simulink model "MdXXArray"  (R2024b)
settings: Solver=FixedStepDiscrete  StartTime=0.0  StopTime=10.0  FixedStep=0.01  RelTol=1e-3
(part 1 of 2)
settings Model: Creator=sn2xws  LastModifiedBy=sn55gm
settings Model: ModifiedHistory=|
  | 2023.8.1 V2.0.0 CR401790 增加模式21-26
  | 2024.7.12 V3.0.0  557模式流程V1.9
  | 2024.10.15 V3.0.1 新增Md57 58
  | 25.6.27 V3.13.0 新增Md62 Md61
settings SolverCC: AlgebraicLoopSolver=TrustRegion
settings DataIOCC: SaveFormat=StructureWithTime  ReturnWorkspaceOutputs=off
settings OptimizationCC: DefaultParameterBehavior=Inlined  EnhancedBackFolding=on  PassReuseOutputArgsAs=Individual arguments  ZeroExternalMemoryAtStartup=off  ZeroInternalMemoryAtStartup=off  OptimizeBlockOrder=speed  DifferentSizesBufferReuse=on  OptimizationCustomize=off  EfficientTunableParamExpr=on
settings DebuggingCC: ParameterTunabilityLossMsg=error  UnconnectedInputMsg=warning  UnconnectedOutputMsg=warning  UnconnectedLineMsg=warning  ArithmeticOperatorsInVariantConditions=warning
settings ModelReferenceCC: EnableRefExpFcnMdlSchedulingChecks=on
settings SFSimCC: MATLABDynamicMemAlloc=off  CustomCodeUndefinedFunction=UseInterfaceOnly
settings RTWCC: Description=AUTOSAR  SystemTargetFile=autosar.tlc  GenCodeOnly=on  TemplateMakefile=ert_default_tmf  GenerateReport=on  IncludeHyperlinkInReport=on  LaunchReport=on  DataTypeReplacement=CDataTypesFixedWidth  GenerateTraceInfo=on  GenerateTraceReport=on  GenerateTraceReportSl=on  GenerateTraceReportSf=on  GenerateTraceReportEml=on  GenerateCodeMetricsReport=on  GPUComputeCapability=3.5
settings CodeAppCC: ForceParamTrailComments=on  IgnoreCustomStorageClasses=off  OperatorAnnotations=on  SimulinkDataObjDesc=on  SFDataObjDesc=on  InsertBlockDesc=on
settings STFCustomTargetCC: TargetLangStandard=C99 (ISO)  MultiwordLength=256  ParMdlRefBuildCompliant=on  CompOptLevelCompliant=on  IncludeMdlTerminateFcn=off  CombineOutputUpdateFcns=on  SuppressErrorStatus=on  ERTCustomFileBanners=on  SupportNonFinite=off  SupportComplex=off  SupportContinuousTime=off  SupportNonInlinedSFcns=off  RemoveResetFunc=on  MATLABClassNameForMDSCustomization=Simulink.SoftwareTarget.ERTCustomization  AutosarCompliant=on  UseToolchainInfoCompliant=on  LookupTableObjectStructAxisOrder=2,1,3,4,...  LUTObjectStructOrderEvenSpacing=Size,Table,Breakpoints  SystemTargetFile=autosar.tlc
settings ERTTargetCC: TargetLangStandard=C99 (ISO)  ConcurrentExecutionCompliant=off  IncludeMdlTerminateFcn=off  SuppressErrorStatus=on  SupportNonFinite=off  SupportComplex=off  ModelStepFunctionPrototypeControlCompliant=off  CPPClassGenCompliant=off  AutosarCompliant=on  LookupTableObjectStructAxisOrder=2,1,3,4,...  LUTObjectStructOrderEvenSpacing=Size,Table,Breakpoints  ERTCustomFileTemplate=example_file_process.tlc  ERTFilePackagingFormat=Compact  BooleanTrueId=TRUE  BooleanFalseId=FALSE  DynamicArrayContainerType=coder::array

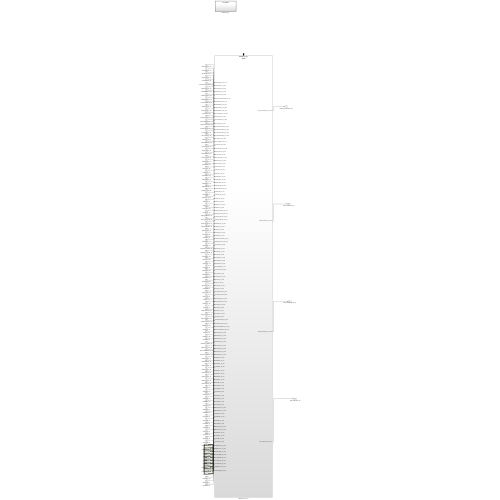
[thumbnail: Simulink's stored preview of the top-level diagram]
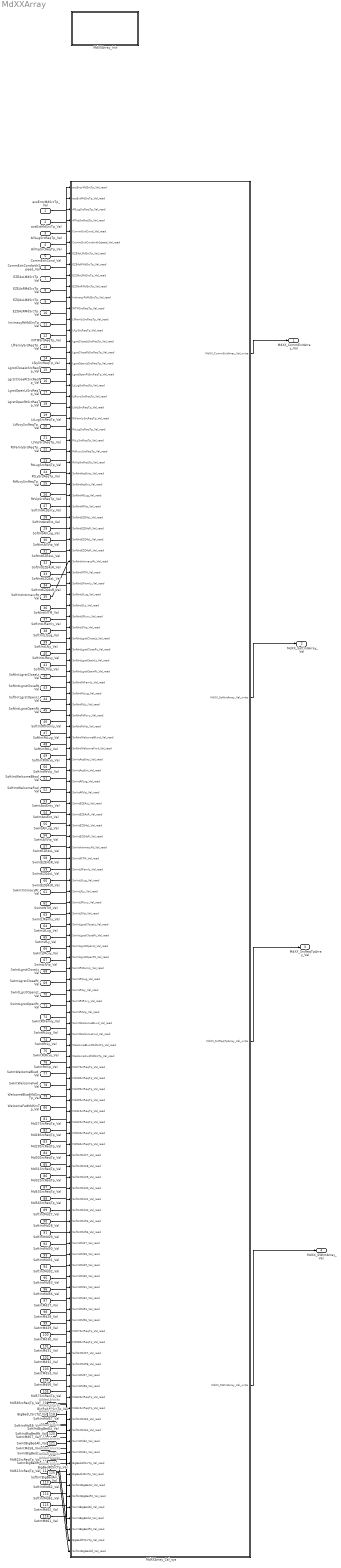
== system MdXXArray ==
  note: Added blocks
  note: Added blocks
  note: Added blocks
  note: Added blocks
  note: Added blocks
  note: Added blocks
  note: Added blocks
  note: Added blocks
  note: Added blocks
  acsEntyMdSrcTp_Val : Inport  OutDataTypeStr=Enum: SrcReqTp1  PortDimensions=1
  acsExtMdSrcTp_Val : Inport  Port=2  OutDataTypeStr=Enum: SrcReqTp1  PortDimensions=1
  AllLugSrcReqTp_Val : Inport  Port=3  OutDataTypeStr=Enum: SrcReqTp1  PortDimensions=1
  AllVipSrcReqTp_Val : Inport  Port=4  OutDataTypeStr=Enum: SrcReqTp1  PortDimensions=1
  CommExitCond_Val : Inport  Port=5  OutDataTypeStr=boolean  PortDimensions=1
  CommExitCondwithSpeed_Val : Inport  Port=6  OutDataTypeStr=boolean  PortDimensions=1
  EZE4sLMdSrcTp_Val : Inport  Port=7  OutDataTypeStr=Enum: SrcReqTp1  PortDimensions=1
  EZE4sRMdSrcTp_Val : Inport  Port=8  OutDataTypeStr=Enum: SrcReqTp1  PortDimensions=1
  EZQ4sLMdSrcTp_Val : Inport  Port=9  OutDataTypeStr=Enum: SrcReqTp1  PortDimensions=1
  EZQ4sRMdSrcTp_Val : Inport  Port=10  OutDataTypeStr=Enum: SrcReqTp1  PortDimensions=1
  IntimacyRtMdSrcTp_Val : Inport  Port=11  OutDataTypeStr=Enum: SrcReqTp1  PortDimensions=1
  INTMSrcReqTp_Val : Inport  Port=12  OutDataTypeStr=Enum: SrcReqTp1  PortDimensions=1
  LfFamlySrcReqTp_Val : Inport  Port=13  OutDataTypeStr=Enum: SrcReqTp1  PortDimensions=1
  LfLySrcReqTp_Val : Inport  Port=14  OutDataTypeStr=Enum: SrcReqTp1  PortDimensions=1
  LgrstCloseLtSrcReqTp_Val : Inport  Port=15  OutDataTypeStr=Enum: SrcReqTp1  PortDimensions=1
  LgrstCloseRtSrcReqTp_Val : Inport  Port=16  OutDataTypeStr=Enum: SrcReqTp1  PortDimensions=1
  LgrstOpenLtSrcReqTp_Val : Inport  Port=17  OutDataTypeStr=Enum: SrcReqTp1  PortDimensions=1
  LgrstOpenRtSrcReqTp_Val : Inport  Port=18  OutDataTypeStr=Enum: SrcReqTp1  PortDimensions=1
  LtLugSrcReqTp_Val : Inport  Port=19  OutDataTypeStr=Enum: SrcReqTp1  PortDimensions=1
  LtRcvySrcReqTp_Val : Inport  Port=20  OutDataTypeStr=Enum: SrcReqTp1  PortDimensions=1
  LtVipSrcReqTp_Val : Inport  Port=21  OutDataTypeStr=Enum: SrcReqTp1  PortDimensions=1
  RtFamlySrcReqTp_Val : Inport  Port=22  OutDataTypeStr=Enum: SrcReqTp1  PortDimensions=1
  RtLugSrcReqTp_Val : Inport  Port=23  OutDataTypeStr=Enum: SrcReqTp1  PortDimensions=1
  RtLySrcReqTp_Val : Inport  Port=24  OutDataTypeStr=Enum: SrcReqTp1  PortDimensions=1
  RtRcvySrcReqTp_Val : Inport  Port=25  OutDataTypeStr=Enum: SrcReqTp1  PortDimensions=1
  RtVipSrcReqTp_Val : Inport  Port=26  OutDataTypeStr=Enum: SrcReqTp1  PortDimensions=1
  SoftIntAcsEnty_Val : Inport  Port=27  OutDataTypeStr=IntEnable  PortDimensions=1
  SoftIntAcsExt_Val : Inport  Port=28  OutDataTypeStr=IntEnable  PortDimensions=1
  SoftIntAllLug_Val : Inport  Port=29  OutDataTypeStr=IntEnable  PortDimensions=1
  SoftIntAllVip_Val : Inport  Port=30  OutDataTypeStr=IntEnable  PortDimensions=1
  SoftIntEZE4sL_Val : Inport  Port=31  OutDataTypeStr=IntEnable  PortDimensions=1
  SoftIntEZE4sR_Val : Inport  Port=32  OutDataTypeStr=IntEnable  PortDimensions=1
  SoftIntEZQ4sL_Val : Inport  Port=33  OutDataTypeStr=IntEnable  PortDimensions=1
  SoftIntEZQ4sR_Val : Inport  Port=34  OutDataTypeStr=IntEnable  PortDimensions=1
  SoftIntIntimacyRt_Val : Inport  Port=35  OutDataTypeStr=IntEnable  PortDimensions=1
  SoftIntINTM_Val : Inport  Port=36  OutDataTypeStr=IntEnable  PortDimensions=1
  SoftIntLfFamly_Val : Inport  Port=37  OutDataTypeStr=IntEnable  PortDimensions=1
  SoftIntLfLug_Val : Inport  Port=38  OutDataTypeStr=IntEnable  PortDimensions=1
  SoftIntLfLy_Val : Inport  Port=39  OutDataTypeStr=IntEnable  PortDimensions=1
  SoftIntLfRcvy_Val : Inport  Port=40  OutDataTypeStr=IntEnable  PortDimensions=1
  SoftIntLfVip_Val : Inport  Port=41  OutDataTypeStr=IntEnable  PortDimensions=1
  SoftIntLgrstCloseLt_Val : Inport  Port=42  OutDataTypeStr=IntEnable  PortDimensions=1
  SoftIntLgrstCloseRt_Val : Inport  Port=43  OutDataTypeStr=IntEnable  PortDimensions=1
  SoftIntLgrstOpenLt_Val : Inport  Port=44  OutDataTypeStr=IntEnable  PortDimensions=1
  SoftIntLgrstOpenRt_Val : Inport  Port=45  OutDataTypeStr=IntEnable  PortDimensions=1
  SoftIntRtFamly_Val : Inport  Port=46  OutDataTypeStr=IntEnable  PortDimensions=1
  SoftIntRtLug_Val : Inport  Port=47  OutDataTypeStr=IntEnable  PortDimensions=1
  SoftIntRtLy_Val : Inport  Port=48  OutDataTypeStr=IntEnable  PortDimensions=1
  SoftIntRtRcvy_Val : Inport  Port=49  OutDataTypeStr=IntEnable  PortDimensions=1
  SoftIntRtVip_Val : Inport  Port=50  OutDataTypeStr=IntEnable  PortDimensions=1
  SoftIntWelcomeBkwd_Val : Inport  Port=51  OutDataTypeStr=IntEnable  PortDimensions=1
  SoftIntWelcomeFwd_Val : Inport  Port=52  OutDataTypeStr=IntEnable  PortDimensions=1
  SwIntAcsEnty_Val : Inport  Port=53  OutDataTypeStr=IntEnable  PortDimensions=1
  SwIntAcsExt_Val : Inport  Port=54  OutDataTypeStr=IntEnable  PortDimensions=1
  SwIntAllLug_Val : Inport  Port=55  OutDataTypeStr=IntEnable  PortDimensions=1
  SwIntAllVip_Val : Inport  Port=56  OutDataTypeStr=IntEnable  PortDimensions=1
  SwIntEZE4sL_Val : Inport  Port=57  OutDataTypeStr=IntEnable  PortDimensions=1
  SwIntEZE4sR_Val : Inport  Port=58  OutDataTypeStr=IntEnable  PortDimensions=1
  SwIntEZQ4sL_Val : Inport  Port=59  OutDataTypeStr=IntEnable  PortDimensions=1
  SwIntEZQ4sR_Val : Inport  Port=60  OutDataTypeStr=IntEnable  PortDimensions=1
  SwIntIntimacyRt_Val : Inport  Port=61  OutDataTypeStr=IntEnable  PortDimensions=1
  SwIntINTM_Val : Inport  Port=62  OutDataTypeStr=IntEnable  PortDimensions=1
  SwIntLfFamly_Val : Inport  Port=63  OutDataTypeStr=IntEnable  PortDimensions=1
  SwIntLfLug_Val : Inport  Port=64  OutDataTypeStr=IntEnable  PortDimensions=1
  SwIntLfLy_Val : Inport  Port=65  OutDataTypeStr=IntEnable  PortDimensions=1
  SwIntLfRcvy_Val : Inport  Port=66  OutDataTypeStr=IntEnable  PortDimensions=1
  SwIntLfVip_Val : Inport  Port=67  OutDataTypeStr=IntEnable  PortDimensions=1
  SwIntLgrstCloseLt_Val : Inport  Port=68  OutDataTypeStr=IntEnable  PortDimensions=1
  SwIntLgrstCloseRt_Val : Inport  Port=69  OutDataTypeStr=IntEnable  PortDimensions=1
  SwIntLgrstOpenLt_Val : Inport  Port=70  OutDataTypeStr=IntEnable  PortDimensions=1
  SwIntLgrstOpenRt_Val : Inport  Port=71  OutDataTypeStr=IntEnable  PortDimensions=1
  SwIntRtFamly_Val : Inport  Port=72  OutDataTypeStr=IntEnable  PortDimensions=1
  SwIntRtLug_Val : Inport  Port=73  OutDataTypeStr=IntEnable  PortDimensions=1
  SwIntRtLy_Val : Inport  Port=74  OutDataTypeStr=IntEnable  PortDimensions=1
  SwIntRtRcvy_Val : Inport  Port=75  OutDataTypeStr=IntEnable  PortDimensions=1
  SwIntRtVip_Val : Inport  Port=76  OutDataTypeStr=IntEnable  PortDimensions=1
  SwIntWelcomeBkwd_Val : Inport  Port=77  OutDataTypeStr=IntEnable  PortDimensions=1
  SwIntWelcomeFwd_Val : Inport  Port=78  OutDataTypeStr=IntEnable  PortDimensions=1
  WelcomeBkwdMdSrcTp_Val : Inport  Port=79  OutDataTypeStr=Enum: SrcReqTp1  PortDimensions=1
  WelcomeFwdMdSrcTp_Val : Inport  Port=80  OutDataTypeStr=Enum: SrcReqTp1  PortDimensions=1
  Md27SrcReqTp_Val : Inport  Port=81  OutDataTypeStr=Enum: SrcReqTp1  PortDimensions=1
  Md28SrcReqTp_Val : Inport  Port=82  OutDataTypeStr=Enum: SrcReqTp1  PortDimensions=1
  Md29SrcReqTp_Val : Inport  Port=83  OutDataTypeStr=Enum: SrcReqTp1  PortDimensions=1
  Md30SrcReqTp_Val : Inport  Port=84  OutDataTypeStr=Enum: SrcReqTp1  PortDimensions=1
  Md31SrcReqTp_Val : Inport  Port=85  OutDataTypeStr=Enum: SrcReqTp1  PortDimensions=1
  Md32SrcReqTp_Val : Inport  Port=86  OutDataTypeStr=Enum: SrcReqTp1  PortDimensions=1
  Md53SrcReqTp_Val : Inport  Port=87  OutDataTypeStr=Enum: SrcReqTp1  PortDimensions=1
  Md56SrcReqTp_Val : Inport  Port=88  OutDataTypeStr=Enum: SrcReqTp1  PortDimensions=1
  SoftIntMd27_Val : Inport  Port=89  OutDataTypeStr=IntEnable  PortDimensions=1
  SoftIntMd28_Val : Inport  Port=90  OutDataTypeStr=IntEnable  PortDimensions=1
  SoftIntMd29_Val : Inport  Port=91  OutDataTypeStr=IntEnable  PortDimensions=1
  SoftIntMd30_Val : Inport  Port=92  OutDataTypeStr=IntEnable  PortDimensions=1
  SoftIntMd31_Val : Inport  Port=93  OutDataTypeStr=IntEnable  PortDimensions=1
  SoftIntMd32_Val : Inport  Port=94  OutDataTypeStr=IntEnable  PortDimensions=1
  SoftIntMd53_Val : Inport  Port=95  OutDataTypeStr=IntEnable  PortDimensions=1
  SoftIntMd56_Val : Inport  Port=96  OutDataTypeStr=IntEnable  PortDimensions=1
  SwIntMd27_Val : Inport  Port=97  OutDataTypeStr=IntEnable  PortDimensions=1
  SwIntMd28_Val : Inport  Port=98  OutDataTypeStr=IntEnable  PortDimensions=1
  SwIntMd29_Val : Inport  Port=99  OutDataTypeStr=IntEnable  PortDimensions=1
  SwIntMd30_Val : Inport  Port=100  OutDataTypeStr=IntEnable  PortDimensions=1
  SwIntMd31_Val : Inport  Port=101  OutDataTypeStr=IntEnable  PortDimensions=1
  SwIntMd32_Val : Inport  Port=102  OutDataTypeStr=IntEnable  PortDimensions=1
  SwIntMd53_Val : Inport  Port=103  OutDataTypeStr=IntEnable  PortDimensions=1
  SwIntMd56_Val : Inport  Port=104  OutDataTypeStr=IntEnable  PortDimensions=1
  Md57SrcReqTp_Val : Inport  Port=105  OutDataTypeStr=Enum: SrcReqTp1  PortDimensions=1
  Md58SrcReqTp_Val : Inport  Port=106  OutDataTypeStr=Enum: SrcReqTp1  PortDimensions=1
  SoftIntMd57_Val : Inport  Port=107  OutDataTypeStr=IntEnable  PortDimensions=1
  SoftIntMd58_Val : Inport  Port=108  OutDataTypeStr=IntEnable  PortDimensions=1
  SwIntMd57_Val : Inport  Port=109  OutDataTypeStr=IntEnable  PortDimensions=1
  SwIntMd58_Val : Inport  Port=110  OutDataTypeStr=IntEnable  PortDimensions=1
  Md62SrcReqTp_Val : Inport  Port=111  OutDataTypeStr=Enum: SrcReqTp1  PortDimensions=1
  Md61SrcReqTp_Val : Inport  Port=112  OutDataTypeStr=Enum: SrcReqTp1  PortDimensions=1
  SoftIntMd62_Val : Inport  Port=113  OutDataTypeStr=IntEnable  PortDimensions=1
  SoftIntMd61_Val : Inport  Port=114  OutDataTypeStr=IntEnable  PortDimensions=1
  SwIntMd62_Val : Inport  Port=115  OutDataTypeStr=IntEnable  PortDimensions=1
  SwIntMd61_Val : Inport  Port=116  OutDataTypeStr=IntEnable  PortDimensions=1
  BigBedAllSrcTp_Val : Inport  Port=117  OutDataTypeStr=Enum: SrcReqTp1  PortDimensions=1
  BigBedLtSrcTp_Val : Inport  Port=118  OutDataTypeStr=Enum: SrcReqTp1  PortDimensions=1
  SoftIntBigBedLt_Val : Inport  Port=119  OutDataTypeStr=IntEnable  PortDimensions=1
  SoftIntBigBedRt_Val : Inport  Port=120  OutDataTypeStr=IntEnable  PortDimensions=1
  SwIntBigBedAll_Val : Inport  Port=121  OutDataTypeStr=IntEnable  PortDimensions=1
  SwIntBigBedLt_Val : Inport  Port=122  OutDataTypeStr=IntEnable  PortDimensions=1
  SwIntBigBedRt_Val : Inport  Port=123  OutDataTypeStr=IntEnable  PortDimensions=1
  BigBedRtSrcTp_Val : Inport  Port=124  OutDataTypeStr=Enum: SrcReqTp1  PortDimensions=1
  SoftIntBigBedAll_Val : Inport  Port=125  OutDataTypeStr=IntEnable  PortDimensions=1
  MdXXArray_Cal_sys : Subsystem
  MdXXArray_Init : Subsystem
  MdXX_CommExitArray_Val : Outport  OutDataTypeStr=boolean  PortDimensions=32  VectorParamsAs1DForOutWhenUnconnected=off
  MdXX_SoftIntArray_Val : Outport  Port=2  OutDataTypeStr=boolean  PortDimensions=32  VectorParamsAs1DForOutWhenUnconnected=off
  MdXX_SrcReqTpArray_Val : Outport  Port=3  OutDataTypeStr=Enum: SrcReqTp1  PortDimensions=32  VectorParamsAs1DForOutWhenUnconnected=off
  MdXX_SWIntArray_Val : Outport  Port=4  OutDataTypeStr=boolean  PortDimensions=32  VectorParamsAs1DForOutWhenUnconnected=off
  wires:
  acsEntyMdSrcTp_Val/1 -> MdXXArray_Cal_sys/1(acsEntyMdSrcTp_Val_read)
  acsExtMdSrcTp_Val/1 -> MdXXArray_Cal_sys/2(acsExtMdSrcTp_Val_read)
  AllLugSrcReqTp_Val/1 -> MdXXArray_Cal_sys/3(AllLugSrcReqTp_Val_read)
  AllVipSrcReqTp_Val/1 -> MdXXArray_Cal_sys/4(AllVipSrcReqTp_Val_read)
  CommExitCond_Val/1 -> MdXXArray_Cal_sys/5(CommExitCond_Val_read)
  CommExitCondwithSpeed_Val/1 -> MdXXArray_Cal_sys/6(CommExitCondwithSpeed_Val_read)
  EZE4sLMdSrcTp_Val/1 -> MdXXArray_Cal_sys/7(EZE4sLMdSrcTp_Val_read)
  EZE4sRMdSrcTp_Val/1 -> MdXXArray_Cal_sys/8(EZE4sRMdSrcTp_Val_read)
  EZQ4sLMdSrcTp_Val/1 -> MdXXArray_Cal_sys/9(EZQ4sLMdSrcTp_Val_read)
  EZQ4sRMdSrcTp_Val/1 -> MdXXArray_Cal_sys/10(EZQ4sRMdSrcTp_Val_read)
  IntimacyRtMdSrcTp_Val/1 -> MdXXArray_Cal_sys/11(IntimacyRtMdSrcTp_Val_read)
  INTMSrcReqTp_Val/1 -> MdXXArray_Cal_sys/12(INTMSrcReqTp_Val_read)
  LfFamlySrcReqTp_Val/1 -> MdXXArray_Cal_sys/13(LfFamlySrcReqTp_Val_read)
  LfLySrcReqTp_Val/1 -> MdXXArray_Cal_sys/14(LfLySrcReqTp_Val_read)
  LgrstCloseLtSrcReqTp_Val/1 -> MdXXArray_Cal_sys/15(LgrstCloseLtSrcReqTp_Val_read)
  LgrstCloseRtSrcReqTp_Val/1 -> MdXXArray_Cal_sys/16(LgrstCloseRtSrcReqTp_Val_read)
  LgrstOpenLtSrcReqTp_Val/1 -> MdXXArray_Cal_sys/17(LgrstOpenLtSrcReqTp_Val_read)
  LgrstOpenRtSrcReqTp_Val/1 -> MdXXArray_Cal_sys/18(LgrstOpenRtSrcReqTp_Val_read)
  LtLugSrcReqTp_Val/1 -> MdXXArray_Cal_sys/19(LtLugSrcReqTp_Val_read)
  LtRcvySrcReqTp_Val/1 -> MdXXArray_Cal_sys/20(LtRcvySrcReqTp_Val_read)
  LtVipSrcReqTp_Val/1 -> MdXXArray_Cal_sys/21(LtVipSrcReqTp_Val_read)
  RtFamlySrcReqTp_Val/1 -> MdXXArray_Cal_sys/22(RtFamlySrcReqTp_Val_read)
  RtLugSrcReqTp_Val/1 -> MdXXArray_Cal_sys/23(RtLugSrcReqTp_Val_read)
  RtLySrcReqTp_Val/1 -> MdXXArray_Cal_sys/24(RtLySrcReqTp_Val_read)
  RtRcvySrcReqTp_Val/1 -> MdXXArray_Cal_sys/25(RtRcvySrcReqTp_Val_read)
  RtVipSrcReqTp_Val/1 -> MdXXArray_Cal_sys/26(RtVipSrcReqTp_Val_read)
  SoftIntAcsEnty_Val/1 -> MdXXArray_Cal_sys/27(SoftIntAcsEnty_Val_read)
  SoftIntAcsExt_Val/1 -> MdXXArray_Cal_sys/28(SoftIntAcsExt_Val_read)
  SoftIntAllLug_Val/1 -> MdXXArray_Cal_sys/29(SoftIntAllLug_Val_read)
  SoftIntAllVip_Val/1 -> MdXXArray_Cal_sys/30(SoftIntAllVip_Val_read)
  SoftIntEZE4sL_Val/1 -> MdXXArray_Cal_sys/31(SoftIntEZE4sL_Val_read)
  SoftIntEZE4sR_Val/1 -> MdXXArray_Cal_sys/32(SoftIntEZE4sR_Val_read)
  SoftIntEZQ4sL_Val/1 -> MdXXArray_Cal_sys/33(SoftIntEZQ4sL_Val_read)
  SoftIntEZQ4sR_Val/1 -> MdXXArray_Cal_sys/34(SoftIntEZQ4sR_Val_read)
  SoftIntIntimacyRt_Val/1 -> MdXXArray_Cal_sys/35(SoftIntIntimacyRt_Val_read)
  SoftIntINTM_Val/1 -> MdXXArray_Cal_sys/36(SoftIntINTM_Val_read)
  SoftIntLfFamly_Val/1 -> MdXXArray_Cal_sys/37(SoftIntLfFamly_Val_read)
  SoftIntLfLug_Val/1 -> MdXXArray_Cal_sys/38(SoftIntLfLug_Val_read)
  SoftIntLfLy_Val/1 -> MdXXArray_Cal_sys/39(SoftIntLfLy_Val_read)
  SoftIntLfRcvy_Val/1 -> MdXXArray_Cal_sys/40(SoftIntLfRcvy_Val_read)
  SoftIntLfVip_Val/1 -> MdXXArray_Cal_sys/41(SoftIntLfVip_Val_read)
  SoftIntLgrstCloseLt_Val/1 -> MdXXArray_Cal_sys/42(SoftIntLgrstCloseLt_Val_read)
  SoftIntLgrstCloseRt_Val/1 -> MdXXArray_Cal_sys/43(SoftIntLgrstCloseRt_Val_read)
  SoftIntLgrstOpenLt_Val/1 -> MdXXArray_Cal_sys/44(SoftIntLgrstOpenLt_Val_read)
  SoftIntLgrstOpenRt_Val/1 -> MdXXArray_Cal_sys/45(SoftIntLgrstOpenRt_Val_read)
  SoftIntRtFamly_Val/1 -> MdXXArray_Cal_sys/46(SoftIntRtFamly_Val_read)
  SoftIntRtLug_Val/1 -> MdXXArray_Cal_sys/47(SoftIntRtLug_Val_read)
  SoftIntRtLy_Val/1 -> MdXXArray_Cal_sys/48(SoftIntRtLy_Val_read)
  SoftIntRtRcvy_Val/1 -> MdXXArray_Cal_sys/49(SoftIntRtRcvy_Val_read)
  SoftIntRtVip_Val/1 -> MdXXArray_Cal_sys/50(SoftIntRtVip_Val_read)
  SoftIntWelcomeBkwd_Val/1 -> MdXXArray_Cal_sys/51(SoftIntWelcomeBkwd_Val_read)
  SoftIntWelcomeFwd_Val/1 -> MdXXArray_Cal_sys/52(SoftIntWelcomeFwd_Val_read)
  SwIntAcsEnty_Val/1 -> MdXXArray_Cal_sys/53(SwIntAcsEnty_Val_read)
  SwIntAcsExt_Val/1 -> MdXXArray_Cal_sys/54(SwIntAcsExt_Val_read)
  SwIntAllLug_Val/1 -> MdXXArray_Cal_sys/55(SwIntAllLug_Val_read)
  SwIntAllVip_Val/1 -> MdXXArray_Cal_sys/56(SwIntAllVip_Val_read)
  SwIntEZE4sL_Val/1 -> MdXXArray_Cal_sys/57(SwIntEZE4sL_Val_read)
  SwIntEZE4sR_Val/1 -> MdXXArray_Cal_sys/58(SwIntEZE4sR_Val_read)
  SwIntEZQ4sL_Val/1 -> MdXXArray_Cal_sys/59(SwIntEZQ4sL_Val_read)
  SwIntEZQ4sR_Val/1 -> MdXXArray_Cal_sys/60(SwIntEZQ4sR_Val_read)
  SwIntIntimacyRt_Val/1 -> MdXXArray_Cal_sys/61(SwIntIntimacyRt_Val_read)
  SwIntINTM_Val/1 -> MdXXArray_Cal_sys/62(SwIntINTM_Val_read)
  SwIntLfFamly_Val/1 -> MdXXArray_Cal_sys/63(SwIntLfFamly_Val_read)
  SwIntLfLug_Val/1 -> MdXXArray_Cal_sys/64(SwIntLfLug_Val_read)
  SwIntLfLy_Val/1 -> MdXXArray_Cal_sys/65(SwIntLfLy_Val_read)
  SwIntLfRcvy_Val/1 -> MdXXArray_Cal_sys/66(SwIntLfRcvy_Val_read)
  SwIntLfVip_Val/1 -> MdXXArray_Cal_sys/67(SwIntLfVip_Val_read)
  SwIntLgrstCloseLt_Val/1 -> MdXXArray_Cal_sys/68(SwIntLgrstCloseLt_Val_read)
  SwIntLgrstCloseRt_Val/1 -> MdXXArray_Cal_sys/69(SwIntLgrstCloseRt_Val_read)
  SwIntLgrstOpenLt_Val/1 -> MdXXArray_Cal_sys/70(SwIntLgrstOpenLt_Val_read)
  SwIntLgrstOpenRt_Val/1 -> MdXXArray_Cal_sys/71(SwIntLgrstOpenRt_Val_read)
  SwIntRtFamly_Val/1 -> MdXXArray_Cal_sys/72(SwIntRtFamly_Val_read)
  SwIntRtLug_Val/1 -> MdXXArray_Cal_sys/73(SwIntRtLug_Val_read)
  SwIntRtLy_Val/1 -> MdXXArray_Cal_sys/74(SwIntRtLy_Val_read)
  SwIntRtRcvy_Val/1 -> MdXXArray_Cal_sys/75(SwIntRtRcvy_Val_read)
  SwIntRtVip_Val/1 -> MdXXArray_Cal_sys/76(SwIntRtVip_Val_read)
  SwIntWelcomeBkwd_Val/1 -> MdXXArray_Cal_sys/77(SwIntWelcomeBkwd_Val_read)
  SwIntWelcomeFwd_Val/1 -> MdXXArray_Cal_sys/78(SwIntWelcomeFwd_Val_read)
  WelcomeBkwdMdSrcTp_Val/1 -> MdXXArray_Cal_sys/79(WelcomeBkwdMdSrcTp_Val_read)
  WelcomeFwdMdSrcTp_Val/1 -> MdXXArray_Cal_sys/80(WelcomeFwdMdSrcTp_Val_read)
  MdXXArray_Cal_sys/1(MdXX_CommExitArray_Val_write) -> MdXX_CommExitArray_Val/1
  MdXXArray_Cal_sys/2(MdXX_SoftIntArray_Val_write) -> MdXX_SoftIntArray_Val/1
  MdXXArray_Cal_sys/3(MdXX_SrcReqTpArray_Val_write) -> MdXX_SrcReqTpArray_Val/1
  MdXXArray_Cal_sys/4(MdXX_SWIntArray_Val_write) -> MdXX_SWIntArray_Val/1
  Md27SrcReqTp_Val/1 -> MdXXArray_Cal_sys/81(Md27SrcReqTp_Val_read)
  Md28SrcReqTp_Val/1 -> MdXXArray_Cal_sys/82(Md28SrcReqTp_Val_read)
  Md29SrcReqTp_Val/1 -> MdXXArray_Cal_sys/83(Md29SrcReqTp_Val_read)
  Md30SrcReqTp_Val/1 -> MdXXArray_Cal_sys/84(Md30SrcReqTp_Val_read)
  Md31SrcReqTp_Val/1 -> MdXXArray_Cal_sys/85(Md31SrcReqTp_Val_read)
  Md32SrcReqTp_Val/1 -> MdXXArray_Cal_sys/86(Md32SrcReqTp_Val_read)
  Md53SrcReqTp_Val/1 -> MdXXArray_Cal_sys/87(Md53SrcReqTp_Val_read)
  Md56SrcReqTp_Val/1 -> MdXXArray_Cal_sys/88(Md56SrcReqTp_Val_read)
  SoftIntMd27_Val/1 -> MdXXArray_Cal_sys/89(SoftIntMd27_Val_read)
  SoftIntMd28_Val/1 -> MdXXArray_Cal_sys/90(SoftIntMd28_Val_read)
  SoftIntMd29_Val/1 -> MdXXArray_Cal_sys/91(SoftIntMd29_Val_read)
  SoftIntMd30_Val/1 -> MdXXArray_Cal_sys/92(SoftIntMd30_Val_read)
  SoftIntMd31_Val/1 -> MdXXArray_Cal_sys/93(SoftIntMd31_Val_read)
  SoftIntMd32_Val/1 -> MdXXArray_Cal_sys/94(SoftIntMd32_Val_read)
  SoftIntMd53_Val/1 -> MdXXArray_Cal_sys/95(SoftIntMd53_Val_read)
  SoftIntMd56_Val/1 -> MdXXArray_Cal_sys/96(SoftIntMd56_Val_read)
  SwIntMd27_Val/1 -> MdXXArray_Cal_sys/97(SwIntMd27_Val_read)
  SwIntMd28_Val/1 -> MdXXArray_Cal_sys/98(SwIntMd28_Val_read)
  SwIntMd29_Val/1 -> MdXXArray_Cal_sys/99(SwIntMd29_Val_read)
  SwIntMd30_Val/1 -> MdXXArray_Cal_sys/100(SwIntMd30_Val_read)
  SwIntMd31_Val/1 -> MdXXArray_Cal_sys/101(SwIntMd31_Val_read)
  SwIntMd32_Val/1 -> MdXXArray_Cal_sys/102(SwIntMd32_Val_read)
  SwIntMd53_Val/1 -> MdXXArray_Cal_sys/103(SwIntMd53_Val_read)
  SwIntMd56_Val/1 -> MdXXArray_Cal_sys/104(SwIntMd56_Val_read)
  Md57SrcReqTp_Val/1 -> MdXXArray_Cal_sys/105(Md57SrcReqTp_Val_read)
  Md58SrcReqTp_Val/1 -> MdXXArray_Cal_sys/106(Md58SrcReqTp_Val_read)
  SoftIntMd57_Val/1 -> MdXXArray_Cal_sys/107(SoftIntMd57_Val_read)
  SoftIntMd58_Val/1 -> MdXXArray_Cal_sys/108(SoftIntMd58_Val_read)
  SwIntMd57_Val/1 -> MdXXArray_Cal_sys/109(SwIntMd57_Val_read)
  SwIntMd58_Val/1 -> MdXXArray_Cal_sys/110(SwIntMd58_Val_read)
  Md62SrcReqTp_Val/1 -> MdXXArray_Cal_sys/111(Md62SrcReqTp_Val_read)
  Md61SrcReqTp_Val/1 -> MdXXArray_Cal_sys/112(Md61SrcReqTp_Val_read)
  SoftIntMd62_Val/1 -> MdXXArray_Cal_sys/113(SoftIntMd62_Val_read)
  SoftIntMd61_Val/1 -> MdXXArray_Cal_sys/114(SoftIntMd61_Val_read)
  SwIntMd62_Val/1 -> MdXXArray_Cal_sys/115(SwIntMd62_Val_read)
  SwIntMd61_Val/1 -> MdXXArray_Cal_sys/116(SwIntMd61_Val_read)
  BigBedAllSrcTp_Val/1 -> MdXXArray_Cal_sys/117(BigBedAllSrcTp_Val_read)
  BigBedLtSrcTp_Val/1 -> MdXXArray_Cal_sys/118(BigBedLtSrcTp_Val_read)
  SoftIntBigBedLt_Val/1 -> MdXXArray_Cal_sys/119(SoftIntBigBedLt_Val_read)
  SoftIntBigBedRt_Val/1 -> MdXXArray_Cal_sys/120(SoftIntBigBedRt_Val_read)
  SwIntBigBedAll_Val/1 -> MdXXArray_Cal_sys/121(SwIntBigBedAll_Val_read)
  SwIntBigBedLt_Val/1 -> MdXXArray_Cal_sys/122(SwIntBigBedLt_Val_read)
  SwIntBigBedRt_Val/1 -> MdXXArray_Cal_sys/123(SwIntBigBedRt_Val_read)
  BigBedRtSrcTp_Val/1 -> MdXXArray_Cal_sys/124(BigBedRtSrcTp_Val_read)
  SoftIntBigBedAll_Val/1 -> MdXXArray_Cal_sys/125(SoftIntBigBedAll_Val_read)

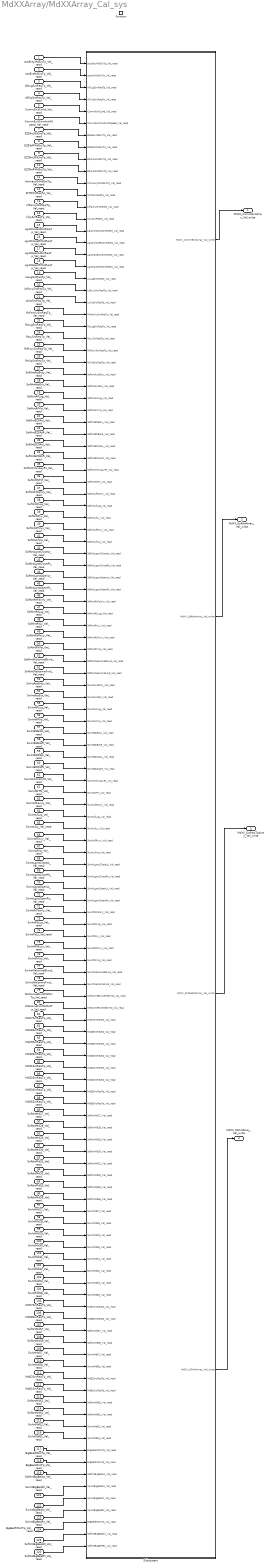
== system MdXXArray/MdXXArray_Cal_sys ==
  acsEntyMdSrcTp_Val_read : Inport
  acsExtMdSrcTp_Val_read : Inport  Port=2
  AllLugSrcReqTp_Val_read : Inport  Port=3
  AllVipSrcReqTp_Val_read : Inport  Port=4
  CommExitCond_Val_read : Inport  Port=5
  CommExitCondwithSpeed_Val_read : Inport  Port=6
  EZE4sLMdSrcTp_Val_read : Inport  Port=7
  EZE4sRMdSrcTp_Val_read : Inport  Port=8
  EZQ4sLMdSrcTp_Val_read : Inport  Port=9
  EZQ4sRMdSrcTp_Val_read : Inport  Port=10
  IntimacyRtMdSrcTp_Val_read : Inport  Port=11
  INTMSrcReqTp_Val_read : Inport  Port=12
  LfFamlySrcReqTp_Val_read : Inport  Port=13
  LfLySrcReqTp_Val_read : Inport  Port=14
  LgrstCloseLtSrcReqTp_Val_read : Inport  Port=15
  LgrstCloseRtSrcReqTp_Val_read : Inport  Port=16
  LgrstOpenLtSrcReqTp_Val_read : Inport  Port=17
  LgrstOpenRtSrcReqTp_Val_read : Inport  Port=18
  LtLugSrcReqTp_Val_read : Inport  Port=19
  LtRcvySrcReqTp_Val_read : Inport  Port=20
  LtVipSrcReqTp_Val_read : Inport  Port=21
  RtFamlySrcReqTp_Val_read : Inport  Port=22
  RtLugSrcReqTp_Val_read : Inport  Port=23
  RtLySrcReqTp_Val_read : Inport  Port=24
  RtRcvySrcReqTp_Val_read : Inport  Port=25
  RtVipSrcReqTp_Val_read : Inport  Port=26
  SoftIntAcsEnty_Val_read : Inport  Port=27
  SoftIntAcsExt_Val_read : Inport  Port=28
  SoftIntAllLug_Val_read : Inport  Port=29
  SoftIntAllVip_Val_read : Inport  Port=30
  SoftIntEZE4sL_Val_read : Inport  Port=31
  SoftIntEZE4sR_Val_read : Inport  Port=32
  SoftIntEZQ4sL_Val_read : Inport  Port=33
  SoftIntEZQ4sR_Val_read : Inport  Port=34
  SoftIntIntimacyRt_Val_read : Inport  Port=35
  SoftIntINTM_Val_read : Inport  Port=36
  SoftIntLfFamly_Val_read : Inport  Port=37
  SoftIntLfLug_Val_read : Inport  Port=38
  SoftIntLfLy_Val_read : Inport  Port=39
  SoftIntLfRcvy_Val_read : Inport  Port=40
  SoftIntLfVip_Val_read : Inport  Port=41
  SoftIntLgrstCloseLt_Val_read : Inport  Port=42
  SoftIntLgrstCloseRt_Val_read : Inport  Port=43
  SoftIntLgrstOpenLt_Val_read : Inport  Port=44
  SoftIntLgrstOpenRt_Val_read : Inport  Port=45
  SoftIntRtFamly_Val_read : Inport  Port=46
  SoftIntRtLug_Val_read : Inport  Port=47
  SoftIntRtLy_Val_read : Inport  Port=48
  SoftIntRtRcvy_Val_read : Inport  Port=49
  SoftIntRtVip_Val_read : Inport  Port=50
  SoftIntWelcomeBkwd_Val_read : Inport  Port=51
  SoftIntWelcomeFwd_Val_read : Inport  Port=52
  SwIntAcsEnty_Val_read : Inport  Port=53
  SwIntAcsExt_Val_read : Inport  Port=54
  SwIntAllLug_Val_read : Inport  Port=55
  SwIntAllVip_Val_read : Inport  Port=56
  SwIntEZE4sL_Val_read : Inport  Port=57
  SwIntEZE4sR_Val_read : Inport  Port=58
  SwIntEZQ4sL_Val_read : Inport  Port=59
  SwIntEZQ4sR_Val_read : Inport  Port=60
  SwIntIntimacyRt_Val_read : Inport  Port=61
  SwIntINTM_Val_read : Inport  Port=62
  SwIntLfFamly_Val_read : Inport  Port=63
  SwIntLfLug_Val_read : Inport  Port=64
  SwIntLfLy_Val_read : Inport  Port=65
  SwIntLfRcvy_Val_read : Inport  Port=66
  SwIntLfVip_Val_read : Inport  Port=67
  SwIntLgrstCloseLt_Val_read : Inport  Port=68
  SwIntLgrstCloseRt_Val_read : Inport  Port=69
  SwIntLgrstOpenLt_Val_read : Inport  Port=70
  SwIntLgrstOpenRt_Val_read : Inport  Port=71
  SwIntRtFamly_Val_read : Inport  Port=72
  SwIntRtLug_Val_read : Inport  Port=73
  SwIntRtLy_Val_read : Inport  Port=74
  SwIntRtRcvy_Val_read : Inport  Port=75
  SwIntRtVip_Val_read : Inport  Port=76
  SwIntWelcomeBkwd_Val_read : Inport  Port=77
  SwIntWelcomeFwd_Val_read : Inport  Port=78
  WelcomeBkwdMdSrcTp_Val_read : Inport  Port=79
  WelcomeFwdMdSrcTp_Val_read : Inport  Port=80
  Md27SrcReqTp_Val_read : Inport  Port=81
  Md28SrcReqTp_Val_read : Inport  Port=82
  Md29SrcReqTp_Val_read : Inport  Port=83
  Md30SrcReqTp_Val_read : Inport  Port=84
  Md31SrcReqTp_Val_read : Inport  Port=85
  Md32SrcReqTp_Val_read : Inport  Port=86
  Md53SrcReqTp_Val_read : Inport  Port=87
  Md56SrcReqTp_Val_read : Inport  Port=88
  SoftIntMd27_Val_read : Inport  Port=89
  SoftIntMd28_Val_read : Inport  Port=90
  SoftIntMd29_Val_read : Inport  Port=91
  SoftIntMd30_Val_read : Inport  Port=92
  SoftIntMd31_Val_read : Inport  Port=93
  SoftIntMd32_Val_read : Inport  Port=94
  SoftIntMd53_Val_read : Inport  Port=95
  SoftIntMd56_Val_read : Inport  Port=96
  SwIntMd27_Val_read : Inport  Port=97
  SwIntMd28_Val_read : Inport  Port=98
  SwIntMd29_Val_read : Inport  Port=99
  SwIntMd30_Val_read : Inport  Port=100
  SwIntMd31_Val_read : Inport  Port=101
  SwIntMd32_Val_read : Inport  Port=102
  SwIntMd53_Val_read : Inport  Port=103
  SwIntMd56_Val_read : Inport  Port=104
  Md57SrcReqTp_Val_read : Inport  Port=105
  Md58SrcReqTp_Val_read : Inport  Port=106
  SoftIntMd57_Val_read : Inport  Port=107
  SoftIntMd58_Val_read : Inport  Port=108
  SwIntMd57_Val_read : Inport  Port=109
  SwIntMd58_Val_read : Inport  Port=110
  Md62SrcReqTp_Val_read : Inport  Port=111
  Md61SrcReqTp_Val_read : Inport  Port=112
  SoftIntMd62_Val_read : Inport  Port=113
  SoftIntMd61_Val_read : Inport  Port=114
  SwIntMd62_Val_read : Inport  Port=115
  SwIntMd61_Val_read : Inport  Port=116
  BigBedAllSrcTp_Val_read : Inport  Port=117
  BigBedLtSrcTp_Val_read : Inport  Port=118
  SoftIntBigBedLt_Val_read : Inport  Port=119
  SoftIntBigBedRt_Val_read : Inport  Port=120
  SwIntBigBedAll_Val_read : Inport  Port=121
  SwIntBigBedLt_Val_read : Inport  Port=122
  SwIntBigBedRt_Val_read : Inport  Port=123
  BigBedRtSrcTp_Val_read : Inport  Port=124
  SoftIntBigBedAll_Val_read : Inport  Port=125
  function : TriggerPort  TriggerType=function-call  IsSimulinkFunction=on  FunctionName=MdXXArray_Cal  VariantControl=(inherit)
  Subsystem : Subsystem
  MdXX_CommExitArray_Val_write : Outport  VectorParamsAs1DForOutWhenUnconnected=off
  MdXX_SoftIntArray_Val_write : Outport  Port=2  VectorParamsAs1DForOutWhenUnconnected=off
  MdXX_SrcReqTpArray_Val_write : Outport  Port=3  VectorParamsAs1DForOutWhenUnconnected=off
  MdXX_SWIntArray_Val_write : Outport  Port=4  VectorParamsAs1DForOutWhenUnconnected=off
  wires:
  acsEntyMdSrcTp_Val_read/1 -> Subsystem/1(acsEntyMdSrcTp_Val_read)
  acsExtMdSrcTp_Val_read/1 -> Subsystem/2(acsExtMdSrcTp_Val_read)
  AllLugSrcReqTp_Val_read/1 -> Subsystem/3(AllLugSrcReqTp_Val_read)
  AllVipSrcReqTp_Val_read/1 -> Subsystem/4(AllVipSrcReqTp_Val_read)
  CommExitCond_Val_read/1 -> Subsystem/5(CommExitCond_Val_read)
  CommExitCondwithSpeed_Val_read/1 -> Subsystem/6(CommExitCondwithSpeed_Val_read)
  EZE4sLMdSrcTp_Val_read/1 -> Subsystem/7(EZE4sLMdSrcTp_Val_read)
  EZE4sRMdSrcTp_Val_read/1 -> Subsystem/8(EZE4sRMdSrcTp_Val_read)
  EZQ4sLMdSrcTp_Val_read/1 -> Subsystem/9(EZQ4sLMdSrcTp_Val_read)
  EZQ4sRMdSrcTp_Val_read/1 -> Subsystem/10(EZQ4sRMdSrcTp_Val_read)
  IntimacyRtMdSrcTp_Val_read/1 -> Subsystem/11(IntimacyRtMdSrcTp_Val_read)
  INTMSrcReqTp_Val_read/1 -> Subsystem/12(INTMSrcReqTp_Val_read)
  LfFamlySrcReqTp_Val_read/1 -> Subsystem/13(LfFamlySrcReqTp_Val_read)
  LfLySrcReqTp_Val_read/1 -> Subsystem/14(LfLySrcReqTp_Val_read)
  LgrstCloseLtSrcReqTp_Val_read/1 -> Subsystem/15(LgrstCloseLtSrcReqTp_Val_read)
  LgrstCloseRtSrcReqTp_Val_read/1 -> Subsystem/16(LgrstCloseRtSrcReqTp_Val_read)
  LgrstOpenLtSrcReqTp_Val_read/1 -> Subsystem/17(LgrstOpenLtSrcReqTp_Val_read)
  LgrstOpenRtSrcReqTp_Val_read/1 -> Subsystem/18(LgrstOpenRtSrcReqTp_Val_read)
  LtLugSrcReqTp_Val_read/1 -> Subsystem/19(LtLugSrcReqTp_Val_read)
  LtRcvySrcReqTp_Val_read/1 -> Subsystem/20(LtRcvySrcReqTp_Val_read)
  LtVipSrcReqTp_Val_read/1 -> Subsystem/21(LtVipSrcReqTp_Val_read)
  RtFamlySrcReqTp_Val_read/1 -> Subsystem/22(RtFamlySrcReqTp_Val_read)
  RtLugSrcReqTp_Val_read/1 -> Subsystem/23(RtLugSrcReqTp_Val_read)
  RtLySrcReqTp_Val_read/1 -> Subsystem/24(RtLySrcReqTp_Val_read)
  RtRcvySrcReqTp_Val_read/1 -> Subsystem/25(RtRcvySrcReqTp_Val_read)
  RtVipSrcReqTp_Val_read/1 -> Subsystem/26(RtVipSrcReqTp_Val_read)
  SoftIntAcsEnty_Val_read/1 -> Subsystem/27(SoftIntAcsEnty_Val_read)
  SoftIntAcsExt_Val_read/1 -> Subsystem/28(SoftIntAcsExt_Val_read)
  SoftIntAllLug_Val_read/1 -> Subsystem/29(SoftIntAllLug_Val_read)
  SoftIntAllVip_Val_read/1 -> Subsystem/30(SoftIntAllVip_Val_read)
  SoftIntEZE4sL_Val_read/1 -> Subsystem/31(SoftIntEZE4sL_Val_read)
  SoftIntEZE4sR_Val_read/1 -> Subsystem/32(SoftIntEZE4sR_Val_read)
  SoftIntEZQ4sL_Val_read/1 -> Subsystem/33(SoftIntEZQ4sL_Val_read)
  SoftIntEZQ4sR_Val_read/1 -> Subsystem/34(SoftIntEZQ4sR_Val_read)
  SoftIntIntimacyRt_Val_read/1 -> Subsystem/35(SoftIntIntimacyRt_Val_read)
  SoftIntINTM_Val_read/1 -> Subsystem/36(SoftIntINTM_Val_read)
  SoftIntLfFamly_Val_read/1 -> Subsystem/37(SoftIntLfFamly_Val_read)
  SoftIntLfLug_Val_read/1 -> Subsystem/38(SoftIntLfLug_Val_read)
  SoftIntLfLy_Val_read/1 -> Subsystem/39(SoftIntLfLy_Val_read)
  SoftIntLfRcvy_Val_read/1 -> Subsystem/40(SoftIntLfRcvy_Val_read)
  SoftIntLfVip_Val_read/1 -> Subsystem/41(SoftIntLfVip_Val_read)
  SoftIntLgrstCloseLt_Val_read/1 -> Subsystem/42(SoftIntLgrstCloseLt_Val_read)
  SoftIntLgrstCloseRt_Val_read/1 -> Subsystem/43(SoftIntLgrstCloseRt_Val_read)
  SoftIntLgrstOpenLt_Val_read/1 -> Subsystem/44(SoftIntLgrstOpenLt_Val_read)
  SoftIntLgrstOpenRt_Val_read/1 -> Subsystem/45(SoftIntLgrstOpenRt_Val_read)
  SoftIntRtFamly_Val_read/1 -> Subsystem/46(SoftIntRtFamly_Val_read)
  SoftIntRtLug_Val_read/1 -> Subsystem/47(SoftIntRtLug_Val_read)
  SoftIntRtLy_Val_read/1 -> Subsystem/48(SoftIntRtLy_Val_read)
  SoftIntRtRcvy_Val_read/1 -> Subsystem/49(SoftIntRtRcvy_Val_read)
  SoftIntRtVip_Val_read/1 -> Subsystem/50(SoftIntRtVip_Val_read)
  SoftIntWelcomeBkwd_Val_read/1 -> Subsystem/51(SoftIntWelcomeBkwd_Val_read)
  SoftIntWelcomeFwd_Val_read/1 -> Subsystem/52(SoftIntWelcomeFwd_Val_read)
  SwIntAcsEnty_Val_read/1 -> Subsystem/53(SwIntAcsEnty_Val_read)
  SwIntAcsExt_Val_read/1 -> Subsystem/54(SwIntAcsExt_Val_read)
  SwIntAllLug_Val_read/1 -> Subsystem/55(SwIntAllLug_Val_read)
  SwIntAllVip_Val_read/1 -> Subsystem/56(SwIntAllVip_Val_read)
  SwIntEZE4sL_Val_read/1 -> Subsystem/57(SwIntEZE4sL_Val_read)
  SwIntEZE4sR_Val_read/1 -> Subsystem/58(SwIntEZE4sR_Val_read)
  SwIntEZQ4sL_Val_read/1 -> Subsystem/59(SwIntEZQ4sL_Val_read)
  SwIntEZQ4sR_Val_read/1 -> Subsystem/60(SwIntEZQ4sR_Val_read)
  SwIntIntimacyRt_Val_read/1 -> Subsystem/61(SwIntIntimacyRt_Val_read)
  SwIntINTM_Val_read/1 -> Subsystem/62(SwIntINTM_Val_read)
  SwIntLfFamly_Val_read/1 -> Subsystem/63(SwIntLfFamly_Val_read)
  SwIntLfLug_Val_read/1 -> Subsystem/64(SwIntLfLug_Val_read)
  SwIntLfLy_Val_read/1 -> Subsystem/65(SwIntLfLy_Val_read)
  SwIntLfRcvy_Val_read/1 -> Subsystem/66(SwIntLfRcvy_Val_read)
  SwIntLfVip_Val_read/1 -> Subsystem/67(SwIntLfVip_Val_read)
  SwIntLgrstCloseLt_Val_read/1 -> Subsystem/68(SwIntLgrstCloseLt_Val_read)
  SwIntLgrstCloseRt_Val_read/1 -> Subsystem/69(SwIntLgrstCloseRt_Val_read)
  SwIntLgrstOpenLt_Val_read/1 -> Subsystem/70(SwIntLgrstOpenLt_Val_read)
  SwIntLgrstOpenRt_Val_read/1 -> Subsystem/71(SwIntLgrstOpenRt_Val_read)
  SwIntRtFamly_Val_read/1 -> Subsystem/72(SwIntRtFamly_Val_read)
  SwIntRtLug_Val_read/1 -> Subsystem/73(SwIntRtLug_Val_read)
  SwIntRtLy_Val_read/1 -> Subsystem/74(SwIntRtLy_Val_read)
  SwIntRtRcvy_Val_read/1 -> Subsystem/75(SwIntRtRcvy_Val_read)
  SwIntRtVip_Val_read/1 -> Subsystem/76(SwIntRtVip_Val_read)
  SwIntWelcomeBkwd_Val_read/1 -> Subsystem/77(SwIntWelcomeBkwd_Val_read)
  SwIntWelcomeFwd_Val_read/1 -> Subsystem/78(SwIntWelcomeFwd_Val_read)
  WelcomeBkwdMdSrcTp_Val_read/1 -> Subsystem/79(WelcomeBkwdMdSrcTp_Val_read)
  WelcomeFwdMdSrcTp_Val_read/1 -> Subsystem/80(WelcomeFwdMdSrcTp_Val_read)
  Subsystem/1(MdXX_CommExitArray_Val_write) -> MdXX_CommExitArray_Val_write/1
  Subsystem/2(MdXX_SoftIntArray_Val_write) -> MdXX_SoftIntArray_Val_write/1
  Subsystem/3(MdXX_SrcReqTpArray_Val_write) -> MdXX_SrcReqTpArray_Val_write/1
  Subsystem/4(MdXX_SWIntArray_Val_write) -> MdXX_SWIntArray_Val_write/1
  SoftIntMd29_Val_read/1 -> Subsystem/91(SoftIntMd29_Val_read)
  SoftIntMd30_Val_read/1 -> Subsystem/92(SoftIntMd30_Val_read)
  SoftIntMd31_Val_read/1 -> Subsystem/93(SoftIntMd31_Val_read)
  SoftIntMd27_Val_read/1 -> Subsystem/89(SoftIntMd27_Val_read)
  SoftIntMd28_Val_read/1 -> Subsystem/90(SoftIntMd28_Val_read)
  SoftIntMd32_Val_read/1 -> Subsystem/94(SoftIntMd32_Val_read)
  SoftIntMd53_Val_read/1 -> Subsystem/95(SoftIntMd53_Val_read)
  Md32SrcReqTp_Val_read/1 -> Subsystem/86(Md32SrcReqTp_Val_read)
  Md53SrcReqTp_Val_read/1 -> Subsystem/87(Md53SrcReqTp_Val_read)
  Md56SrcReqTp_Val_read/1 -> Subsystem/88(Md56SrcReqTp_Val_read)
  SoftIntMd56_Val_read/1 -> Subsystem/96(SoftIntMd56_Val_read)
  SwIntMd27_Val_read/1 -> Subsystem/97(SwIntMd27_Val_read)
  SwIntMd28_Val_read/1 -> Subsystem/98(SwIntMd28_Val_read)
  Md30SrcReqTp_Val_read/1 -> Subsystem/84(Md30SrcReqTp_Val_read)
  Md31SrcReqTp_Val_read/1 -> Subsystem/85(Md31SrcReqTp_Val_read)
  SwIntMd29_Val_read/1 -> Subsystem/99(SwIntMd29_Val_read)
  SwIntMd30_Val_read/1 -> Subsystem/100(SwIntMd30_Val_read)
  Md27SrcReqTp_Val_read/1 -> Subsystem/81(Md27SrcReqTp_Val_read)
  Md28SrcReqTp_Val_read/1 -> Subsystem/82(Md28SrcReqTp_Val_read)
  Md29SrcReqTp_Val_read/1 -> Subsystem/83(Md29SrcReqTp_Val_read)
  SwIntMd31_Val_read/1 -> Subsystem/101(SwIntMd31_Val_read)
  SwIntMd32_Val_read/1 -> Subsystem/102(SwIntMd32_Val_read)
  SwIntMd53_Val_read/1 -> Subsystem/103(SwIntMd53_Val_read)
  SwIntMd56_Val_read/1 -> Subsystem/104(SwIntMd56_Val_read)
  Md57SrcReqTp_Val_read/1 -> Subsystem/105(Md57SrcReqTp_Val_read)
  Md58SrcReqTp_Val_read/1 -> Subsystem/106(Md58SrcReqTp_Val_read)
  SoftIntMd57_Val_read/1 -> Subsystem/107(SoftIntMd57_Val_read)
  SoftIntMd58_Val_read/1 -> Subsystem/108(SoftIntMd58_Val_read)
  SwIntMd57_Val_read/1 -> Subsystem/109(SwIntMd57_Val_read)
  SwIntMd58_Val_read/1 -> Subsystem/110(SwIntMd58_Val_read)
  Md62SrcReqTp_Val_read/1 -> Subsystem/111(Md62SrcReqTp_Val_read)
  Md61SrcReqTp_Val_read/1 -> Subsystem/112(Md61SrcReqTp_Val_read)
  SoftIntMd62_Val_read/1 -> Subsystem/113(SoftIntMd62_Val_read)
  SoftIntMd61_Val_read/1 -> Subsystem/114(SoftIntMd61_Val_read)
  SwIntMd62_Val_read/1 -> Subsystem/115(SwIntMd62_Val_read)
  SwIntMd61_Val_read/1 -> Subsystem/116(SwIntMd61_Val_read)
  BigBedAllSrcTp_Val_read/1 -> Subsystem/117(BigBedAllSrcTp_Val_read)
  BigBedLtSrcTp_Val_read/1 -> Subsystem/118(BigBedLtSrcTp_Val_read)
  SoftIntBigBedLt_Val_read/1 -> Subsystem/119(SoftIntBigBedLt_Val_read)
  SoftIntBigBedRt_Val_read/1 -> Subsystem/125(SoftIntBigBedRt_Val_read)
  SwIntBigBedAll_Val_read/1 -> Subsystem/120(SwIntBigBedAll_Val_read)
  SwIntBigBedLt_Val_read/1 -> Subsystem/121(SwIntBigBedLt_Val_read)
  SwIntBigBedRt_Val_read/1 -> Subsystem/122(SwIntBigBedRt_Val_read)
  BigBedRtSrcTp_Val_read/1 -> Subsystem/123(BigBedRtSrcTp_Val_read)
  SoftIntBigBedAll_Val_read/1 -> Subsystem/124(SoftIntBigBedAll_Val_read)

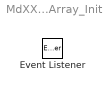
== system MdXXArray/MdXXArray_Init ==
  Event Listener : EventListener  EventName=reset
